simulink model "AFDNFSmodelSPA"  (R2017b)
settings: Solver=ode45  StartTime=0.0  StopTime=1400  FixedStep=1e-3  RelTol=1e-8  EnableMultiTasking=on
PostLoadFcn:
  | run('Methods/NFSOnLoad');
InitFcn:
  | run('Methods/AFDSimInit')
StopFcn:
  | run('Methods/NFSOnLoad');
values from neighbouring files (symbols this model uses):
  nfs = TransferFunction('Plot','true')    [Main.m]    (also in NFSDatabase.sldd = SI
                Imperial
                28184.4409185639)
undefined symbols (not defined in the file or in its folder): Continuous, desired, Earth, F, K_lat, K_long, Kobsvlat, Kobsvlong, lat, latsys, Light, long, longsys, MIL, Newton, Raphson, sigbuilder_block, Time, WGS84
libraries: simulink x6, aerolibtransform2 x2, aerolibwind2 x2, ModelsLibrary x1, ctrlSharedLib x1, sharedutil x1
(part 2 of 4)

== system AFDNFSmodelSPA/Navigation & Sensor System/Navigation Model/01-Test Model/Initialization ==
  Constant4 : Constant  Value=nfs.crusevelvec
  Constant6 : Constant  Value=nfs.angularvel0
  Constant7 : Constant  Value=nfs.attitude0
  Constant8 : Constant  Value=nfs.initialpos
  Reshape{4,6..8} (4 alike) : Reshape  OutputDimensionality=Column vector (2-D)
  Initial Linear Velocity Vector : Outport
  Initial Angular Velocity Vector : Outport  Port=2
  Initial Euler Angles : Outport  Port=3
  Initial Location (NED) : Outport  Port=4
  wires:
  Constant4/1 -> Reshape4/1
  Constant6/1 -> Reshape6/1
  Constant7/1 -> Reshape7/1
  Constant8/1 -> Reshape8/1
  Reshape4/1 -> Initial Linear Velocity Vector/1
  Reshape6/1 -> Initial Angular Velocity Vector/1
  Reshape7/1 -> Initial Euler Angles/1
  Reshape8/1 -> Initial Location (NED)/1

== system AFDNFSmodelSPA/Navigation & Sensor System/Navigation Model/01-Test Model/Navigation Model - Simple ==
  Linear Acceleration (Body) : Inport
  Angular Acceleration (Body) : Inport  Port=2
  Initial Linear Velocity Vector : Inport  Port=3
  Initial Angular Velocity Vector : Inport  Port=4
  Initial Euler Angles : Inport  Port=5
  Initial Location (NED) : Inport  Port=6
  Angular Velocity Integrator (Body) : Integrator  InitialConditionSource=external  InitialCondition=nfs.angularvel0
  Euler angles & Direction Cosine Using Quaternions : Subsystem
  Linear Velocity Integrator (Body) : Integrator  InitialConditionSource=external  InitialCondition=nfs.crusevelvec  ContinuousStateAttributes='BodyVelocity'
  Saturation1 : Saturate  UpperLimit=500  LowerLimit=-500
  Saturation2 : Saturate  UpperLimit=500  LowerLimit=-500
  Linear Velocity (Body) Measured : Outport
  Angular Velocity (Body) Measured : Outport  Port=2
  Euler Angles Measured : Outport  Port=3
  Position (NED) Measured : Outport  Port=4
  Velocity (NED) Measured : Outport  Port=5
  T_BI Measured : Outport  Port=6
  wires:
  Initial Euler Angles/1 -> Euler angles & Direction Cosine Using Quaternions/2(Initial Euler Angles)
  Initial Location (NED)/1 -> Euler angles & Direction Cosine Using Quaternions/3(Initial Location (NED))
  Linear Acceleration (Body)/1 -> Linear Velocity Integrator (Body)/1
  Euler angles & Direction Cosine Using Quaternions/1(Direction Cosine Matrix (T_BI)) -> T_BI Measured/1
  Euler angles & Direction Cosine Using Quaternions/2(Euler Angles) -> Euler Angles Measured/1
  Euler angles & Direction Cosine Using Quaternions/4(Velocity (NED)) -> Velocity (NED) Measured/1
  Saturation1/1 -> Euler angles & Direction Cosine Using Quaternions/1(Linear Velocity), Linear Velocity (Body) Measured/1
  Angular Acceleration (Body)/1 -> Angular Velocity Integrator (Body)/1
  Initial Linear Velocity Vector/1 -> Linear Velocity Integrator (Body)/2
  Euler angles & Direction Cosine Using Quaternions/3(Position (NED)) -> Position (NED) Measured/1
  Linear Velocity Integrator (Body)/1 -> Saturation1/1  "uvw"
  Angular Velocity Integrator (Body)/1 -> Saturation2/1  "pqr"
  Saturation2/1 -> Euler angles & Direction Cosine Using Quaternions/4(Angular Velocities), Angular Velocity (Body) Measured/1
  Initial Angular Velocity Vector/1 -> Angular Velocity Integrator (Body)/2

== system AFDNFSmodelSPA/Nonlinear Flight Simulator/6DoF Nonlinear Flight Equations of Motion (Rigid Body)/AngularAcceleration(Omegadot)/Cross Product ==
  A : Inport
  B : Inport  Port=2
  "A " : InportShadow
  "B " : InportShadow  Port=2
  Subsystem2 : Subsystem
  Subsystem3 : Subsystem
  Sum : Sum  Inputs=+|-  SaturateOnIntegerOverflow=on  InputSameDT=on  OutDataTypeStr=Inherit: Same as first input
  C : Outport
  wires:
  Subsystem3/1(Out2) -> Sum/2
  Subsystem2/1(Out1) -> Sum/1
  A/1 -> Subsystem2/1(A)
  B/1 -> Subsystem2/2(B)
  Sum/1 -> C/1
  "A "/1 -> Subsystem3/1(A)
  "B "/1 -> Subsystem3/2(B)

== system AFDNFSmodelSPA/Nonlinear Flight Simulator/6DoF Nonlinear Flight Equations of Motion (Rigid Body)/Euler angles & Direction Cosine/Euler angles Calculation ==
  Angular Velocities : Inport  PortDimensions=[3,1]
  Euler Angles : Inport  Port=2
  Mux1 : Mux  Inputs=[3 3 3]
  Mux2 : Mux  Inputs=3
  phidot : Fcn  Expr=u[1]+(u[2]*u[4]+u[3]*u[7])*(u[5]/u[8])
  psidot : Fcn  Expr=(u[2]*u[4]+u[3]*u[7])/u[8]
  sincos : Trigonometry  Operator=sincos
  thetadot : Fcn  Expr=u[2]*u[7]-u[3]*u[4]
  Euler Rates : Outport  PortDimensions=[3,1]  InitialOutput=0
  wires:
  sincos/2 -> Mux1/3
  sincos/1 -> Mux1/2
  Mux2/1 -> Euler Rates/1
  phidot/1 -> Mux2/1
  thetadot/1 -> Mux2/2
  psidot/1 -> Mux2/3
  Euler Angles/1 -> sincos/1
  Angular Velocities/1 -> Mux1/1
  Mux1/1 -> psidot/1, phidot/1, thetadot/1

== system AFDNFSmodelSPA/Nonlinear Flight Simulator/6DoF Nonlinear Flight Equations of Motion (Rigid Body)/Euler angles & Direction Cosine/If Action Subsystem ==
  Simulation Termination : Inport
  Action Port : ActionPort  ActionType=then
  Stop Simulation : Stop
  wires:
  Simulation Termination/1 -> Stop Simulation/1

== system AFDNFSmodelSPA/Nonlinear Flight Simulator/6DoF Nonlinear Flight Equations of Motion (Rigid Body)/Euler angles & Direction Cosine/Rotation Angles to DCM ==
  "[R1,R2,R3]" : Inport  PortDimensions=3
  Create 3x3 Matrix : sharedutil/Create 3x3 Matrix
  Fcn11 : Fcn  Expr=u(5)*u(4)
  Fcn12 : Fcn  Expr=u(5)*u(1)
  Fcn13 : Fcn  Expr=-u(2)
  Fcn21 : Fcn  Expr=u(3)*u(2)*u(4) - u(6)*u(1)
  Fcn22 : Fcn  Expr=u(3)*u(2)*u(1) + u(6)*u(4)
  Fcn23 : Fcn  Expr=u(3)*u(5)
  Fcn31 : Fcn  Expr=u(6)*u(2)*u(4) + u(3)*u(1)
  Fcn32 : Fcn  Expr=u(6)*u(2)*u(1) - u(3)*u(4)
  Fcn33 : Fcn  Expr=u(6)*u(5)
  Mux : Mux  Inputs=2
  sincos1 : Trigonometry  Operator=sincos
  DCM : Outport  PortDimensions=[3,3]
  wires:
  "[R1,R2,R3]"/1 -> sincos1/1
  Create 3x3 Matrix/1 -> DCM/1
  sincos1/1 -> Mux/1
  sincos1/2 -> Mux/2
  Mux/1 -> Fcn32/1, Fcn33/1, Fcn31/1, Fcn23/1, Fcn22/1, Fcn11/1, Fcn12/1, Fcn13/1, Fcn21/1
  Fcn11/1 -> Create 3x3 Matrix/1
  Fcn12/1 -> Create 3x3 Matrix/2
  Fcn13/1 -> Create 3x3 Matrix/3
  Fcn21/1 -> Create 3x3 Matrix/4
  Fcn31/1 -> Create 3x3 Matrix/7
  Fcn22/1 -> Create 3x3 Matrix/5
  Fcn23/1 -> Create 3x3 Matrix/6
  Fcn32/1 -> Create 3x3 Matrix/8
  Fcn33/1 -> Create 3x3 Matrix/9

== system AFDNFSmodelSPA/Nonlinear Flight Simulator/6DoF Nonlinear Flight Equations of Motion (Rigid Body)/Euler angles & Direction Cosine/Transform from Body to Inertial axes ==
  Transformation Matrix : Inport
  Position Vector : Inport  Port=2
  Product : Product  Multiplication=Matrix(*)  SaturateOnIntegerOverflow=on  InputSameDT=on  OutDataTypeStr=Inherit: Same as first input
  Reshape1 : Reshape  OutputDimensionality=Column vector (2-D)
  Reshape2 : Reshape
  Ve : Outport
  wires:
  Reshape2/1 -> Ve/1
  Reshape1/1 -> Product/2
  Position Vector/1 -> Reshape1/1
  Transformation Matrix/1 -> Product/1
  Product/1 -> Reshape2/1

== system AFDNFSmodelSPA/Nonlinear Flight Simulator/6DoF Nonlinear Flight Equations of Motion (Rigid Body)/Linear Acceleration(Vdot)/Cross Product ==
  A : Inport
  B : Inport  Port=2
  "A " : InportShadow
  "B " : InportShadow  Port=2
  Subsystem2 : Subsystem
  Subsystem3 : Subsystem
  Sum : Sum  Inputs=+|-  SaturateOnIntegerOverflow=on  InputSameDT=on  OutDataTypeStr=Inherit: Same as first input
  C : Outport
  wires:
  Subsystem3/1(Out2) -> Sum/2
  Subsystem2/1(Out1) -> Sum/1
  A/1 -> Subsystem2/1(A)
  B/1 -> Subsystem2/2(B)
  Sum/1 -> C/1
  "A "/1 -> Subsystem3/1(A)
  "B "/1 -> Subsystem3/2(B)

== system AFDNFSmodelSPA/Nonlinear Flight Simulator/Forces and Moments/Aerodynamic Forces and /Aero Attributes ==
  Linear Velocity (Body) : Inport  PortDimensions=[3,1]
  Altitude : Inport  Port=2
  Beta Saturation : Saturate  UpperLimit=5*pi/11  LowerLimit=-5*pi/11
  Beta Saturation1 : Saturate  UpperLimit=1  LowerLimit=-1
  Demux1 : Demux  Outputs=3
  Derivative1 : Derivative
  Derivative2 : Derivative
  Dynamic Pressure Calc : Subsystem
  Gain : Gain  Gain=0
  Gain1 : Gain
  Linear Velocity (Body)1 : InportShadow  PortDimensions=[3,1]
  Reshape13 : Reshape
  Scope : Scope
  Subsystem : Subsystem
  Trigonometric Function2 : Trigonometry  Operator=atan
  Trigonometric Function3 : Trigonometry  Operator=asin
  Velocity Magnitude : Subsystem
  w/u1 : Product  Inputs=/*  SaturateOnIntegerOverflow=on  InputSameDT=on  OutDataTypeStr=Inherit: Same as first input
  w/u2 : Product  Inputs=*/  SaturateOnIntegerOverflow=on  InputSameDT=on  OutDataTypeStr=Inherit: Same as first input
  w/u3 : Product  Inputs=*/  SaturateOnIntegerOverflow=on  InputSameDT=on  OutDataTypeStr=Inherit: Same as first input
  Alpha : Outport
  Beta : Outport  Port=2
  Dynamic Pressure : Outport  Port=3
  Alphadot : Outport  Port=4
  Betadot : Outport  Port=5
  Mach : Outport  Port=6
  wires:
  Beta Saturation1/1 -> Gain1/1
  Subsystem/2(Air Density) -> Dynamic Pressure Calc/1(Air Density)
  Subsystem/1(Speed of Sound) -> w/u3/2
  Velocity Magnitude/1(Velocity Magnitude) -> w/u3/1, w/u2/2
  Reshape13/1 -> Mach/1
  Derivative2/1 -> Gain/1  "Betadot"
  Beta Saturation/1 -> Beta/1
  Derivative1/1 -> Beta Saturation1/1
  Dynamic Pressure Calc/1(Dynamic Pressure) -> Dynamic Pressure/1
  Linear Velocity (Body)1/1 -> Dynamic Pressure Calc/2(Linear Velocity (Body))
  Altitude/1 -> Subsystem/1(Height)
  w/u3/1 -> Reshape13/1
  Trigonometric Function3/1 -> Beta Saturation/1, Derivative2/1
  Trigonometric Function2/1 -> Derivative1/1, Scope/1, Alpha/1
  w/u2/1 -> Trigonometric Function3/1
  w/u1/1 -> Trigonometric Function2/1
  Demux1/3 -> w/u1/2  "W"
  Demux1/2 -> w/u2/1  "V"
  Demux1/1 -> w/u1/1  "U"
  Linear Velocity (Body)/1 -> Velocity Magnitude/1(Velocity), Demux1/1
  Gain/1 -> Betadot/1
  Gain1/1 -> Alphadot/1

== system AFDNFSmodelSPA/Nonlinear Flight Simulator/Forces and Moments/Aerodynamic Forces and /Energy Analysis1 ==
  Dynamic Pressure : Inport
  Control : Inport  Port=2
  Linear Vel Body : Inport  Port=3
  Angular Vel Body : Inport  Port=4
  Alpha : Inport  Port=5
  Alpha_dot : Inport  Port=6
  Beta : Inport  Port=7
  Beta_dot : Inport  Port=8
  Angular Vel Body0 : InportShadow  Port=4
  Constant{1..2,5,8} (4 alike) : Constant  Value=0
  Constant3 : Constant  Value=ae.refarea
  Constant4 : Constant  Value=ae.span
  Constant6 : Constant  Value=ae.refarea
  Constant9 : Constant  Value=ae.meanchord
  Control3 : InportShadow  Port=2
  Demux1 : Demux
  Demux2 : Demux
  Dynamic Pressure2 : InportShadow
  Lateral-Directional1 : Subsystem
  Linear Vel Body2 : InportShadow  Port=3
  Longitudinal1 : Subsystem
  Lift : Outport
  Drag : Outport  Port=2
  Y Moment : Outport  Port=3
  Side Force : Outport  Port=4
  X Moment : Outport  Port=5
  Z Moment : Outport  Port=6
  wires:
  Lateral-Directional1/1(fy) -> Side Force/1
  Lateral-Directional1/2(l) -> X Moment/1
  Lateral-Directional1/3(n) -> Z Moment/1
  Longitudinal1/2(m) -> Y Moment/1
  Longitudinal1/1(D) -> Drag/1
  Longitudinal1/3(L) -> Lift/1
  Dynamic Pressure/1 -> Lateral-Directional1/1(Dynamic Pressure)
  Constant3/1 -> Lateral-Directional1/2(S)
  Linear Vel Body/1 -> Lateral-Directional1/4(Linear Vel Body)
  Angular Vel Body0/1 -> Lateral-Directional1/5(Angular Vel Body)
  Constant5/1 -> Lateral-Directional1/13(iH)
  Constant4/1 -> Lateral-Directional1/3(b)
  Beta/1 -> Lateral-Directional1/6(Beta)
  Beta_dot/1 -> Lateral-Directional1/7(Beta_dot)
  Demux1/1 -> Lateral-Directional1/8(DeltaElevator)
  Demux1/2 -> Lateral-Directional1/9(DeltaFlap)
  Demux1/4 -> Lateral-Directional1/11(DeltaRudder)
  Demux1/3 -> Lateral-Directional1/10(DeltaAileron)
  Constant1/1 -> Lateral-Directional1/12(DeltaThrust)
  Control/1 -> Demux1/1
  Constant6/1 -> Longitudinal1/2(S)
  Alpha/1 -> Longitudinal1/6(Alpha)
  Angular Vel Body/1 -> Longitudinal1/4(Angular Vel)
  Dynamic Pressure2/1 -> Longitudinal1/1(Dynamic Pressure)
  Linear Vel Body2/1 -> Longitudinal1/3(Linear Vel Body)
  Constant9/1 -> Longitudinal1/5(c_bar)
  Alpha_dot/1 -> Longitudinal1/7(Alpha_dot)
  Constant8/1 -> Longitudinal1/13(iH)
  Constant2/1 -> Longitudinal1/12(Delta_Thrust)
  Demux2/4 -> Longitudinal1/11(DeltaRudder)
  Demux2/2 -> Longitudinal1/9(DeltaFlap)
  Demux2/3 -> Longitudinal1/10(DeltaAileron)
  Demux2/1 -> Longitudinal1/8(DeltaElevator)
  Control3/1 -> Demux2/1

== system AFDNFSmodelSPA/Nonlinear Flight Simulator/Forces and Moments/Aerodynamic Forces and /Forces ==
  Linear Velocity : Inport  PortDimensions=[3,1]
  Alpha : Inport  Port=2  PortDimensions=1
  Beta : Inport  Port=3
  Angular Velocity : Inport  Port=4  PortDimensions=[3,1]
  Control : Inport  Port=5  PortDimensions=[4,1]
  Dynamic Pressure : Inport  Port=6  PortDimensions=[1,1]
  Alphadot : Inport  Port=7  PortDimensions=1
  Mach : Inport  Port=8
  Aerodynamic Forces : Subsystem
  Alpha1 : InportShadow  Port=2  PortDimensions=1
  Beta1 : InportShadow  Port=3
  Force Coefficients Calculator : Subsystem
  Aerodynamic Forces (Body) : Outport
  wires:
  Aerodynamic Forces/1(Aerodynamic Forces) -> Aerodynamic Forces (Body)/1
  Control/1 -> Force Coefficients Calculator/5(Control)
  Angular Velocity/1 -> Force Coefficients Calculator/4(Angular Velocity)
  Alphadot/1 -> Force Coefficients Calculator/6(Alphadot)
  Mach/1 -> Force Coefficients Calculator/7(Mach)
  Linear Velocity/1 -> Force Coefficients Calculator/1(Linear Velocity)
  Alpha/1 -> Force Coefficients Calculator/2(Alpha)
  Beta/1 -> Force Coefficients Calculator/3(Beta)
  Force Coefficients Calculator/1(CL) -> Aerodynamic Forces/1(CL)
  Force Coefficients Calculator/2(CD) -> Aerodynamic Forces/2(CD)
  Force Coefficients Calculator/3(CY) -> Aerodynamic Forces/3(CY)
  Alpha1/1 -> Aerodynamic Forces/5(Alpha)
  Dynamic Pressure/1 -> Aerodynamic Forces/4(Dynamic Pressure)
  Beta1/1 -> Aerodynamic Forces/6(Beta)

== system AFDNFSmodelSPA/Nonlinear Flight Simulator/Forces and Moments/Aerodynamic Forces and /Moments ==
  Linear Velocity : Inport  PortDimensions=[3,1]
  Alpha : Inport  Port=2
  Beta : Inport  Port=3
  Angular Velocity : Inport  Port=4  PortDimensions=[3,1]
  Control : Inport  Port=5
  Dynamic Pressure : Inport  Port=6
  Alphadot : Inport  Port=7
  Mach : Inport  Port=8
  "Aerodynamic Moment " : Subsystem
  Alpha1 : InportShadow  Port=2
  Beta1 : InportShadow  Port=3
  Beta2 : InportShadow  Port=3
  Demux1 : Demux  Outputs=3
  Demux2 : Demux
  Linear Velocity1 : InportShadow  PortDimensions=[3,1]
  Linear Velocity2 : InportShadow  PortDimensions=[3,1]
  Pitch Moment Coefficient : Subsystem
  Roll Moment Coefficient : Subsystem
  Yaw Moment Coefficient : Subsystem
  Aerodynamic Moments (Body) : Outport
  wires:
  Demux2/2 -> Pitch Moment Coefficient/5(DeltaFlap)
  Demux2/1 -> Pitch Moment Coefficient/4(DeltaElevator)
  Demux2/4 -> Yaw Moment Coefficient/6(DeltaRudder), Roll Moment Coefficient/6(DeltaRudder)
  Demux2/3 -> Yaw Moment Coefficient/5(DeltaAileron), Roll Moment Coefficient/5(DeltaAileron)
  Control/1 -> Demux2/1
  Mach/1 -> Pitch Moment Coefficient/7(Mach)
  Alphadot/1 -> Pitch Moment Coefficient/6(Alphadot)
  Demux1/2 -> Pitch Moment Coefficient/3(Q)
  Demux1/3 -> Yaw Moment Coefficient/4(R), Roll Moment Coefficient/4(R)
  Demux1/1 -> Yaw Moment Coefficient/3(P), Roll Moment Coefficient/3(P)
  Angular Velocity/1 -> Demux1/1
  Beta1/1 -> Yaw Moment Coefficient/2(beta)
  Beta/1 -> Roll Moment Coefficient/2(Beta)
  Alpha/1 -> Pitch Moment Coefficient/2(Alpha)
  Dynamic Pressure/1 -> "Aerodynamic Moment "/4(Dynamic Pressure)
  Linear Velocity2/1 -> Yaw Moment Coefficient/1(Linear Velocity)
  Linear Velocity1/1 -> Pitch Moment Coefficient/1(Linear Velocity)
  Linear Velocity/1 -> Roll Moment Coefficient/1(Linear Velocity)
  "Aerodynamic Moment "/1(Aerodynamic Moments) -> Aerodynamic Moments (Body)/1
  Yaw Moment Coefficient/1(Cn) -> "Aerodynamic Moment "/3(Cn)
  Pitch Moment Coefficient/1(Cm) -> "Aerodynamic Moment "/2(Cm)
  Roll Moment Coefficient/1(Cl) -> "Aerodynamic Moment "/1(Cl)
  Alpha1/1 -> "Aerodynamic Moment "/5(Alpha)
  Beta2/1 -> "Aerodynamic Moment "/6(Beta)

== system AFDNFSmodelSPA/Nonlinear Flight Simulator/Forces and Moments/Aerodynamic Forces and /Turbulence ==
  Linear Velocity : Inport  PortDimensions=[3,1]
  Angular Velocity : Inport  Port=2  PortDimensions=[3,1]
  Altitude : Inport  Port=3  PortDimensions=1
  DCM : Inport  Port=4  PortDimensions=[3,3]
  Bus Creator : BusCreator  Inputs=4
  Turbulence Model : Subsystem  Variant=on
  Turbulent Velocity : Outport
  wires:
  Linear Velocity/1 -> Bus Creator/1  "Linear Velocity"
  Altitude/1 -> Bus Creator/3  "Altitude"
  DCM/1 -> Bus Creator/4  "DCM"
  Bus Creator/1 -> Turbulence Model/1(In)
  Angular Velocity/1 -> Bus Creator/2  "Angular Velocity"
  Turbulence Model/1(Out) -> Turbulent Velocity/1

== system AFDNFSmodelSPA/Nonlinear Flight Simulator/Forces and Moments/Thrust/Signal Builder ==
  Demux : Demux  Tag=STV Demux  Outputs=1
  FromWs : FromWorkspace  Tag=STV FromWs  VariableName=tuvar  SampleTime=0
      SigBuilderData=|
      | common.afterFinalStr = 'Extrapolate'
      | common.sampleTime = 0
      | dataSet.timeRange = [0 1200]
      | dataSet.name = 'Thrust Deviation'
      | sbobj.Groups.Name = 'Thrust Deviation'
      | sbobj.Groups.Signals.Name = 'ThrustDeviation'
      | sbobj.Groups.Signals.XData = [0 10 10 12 12 1200]
      | sbobj.Groups.Signals.YData = [1 1 1.05 1.05 1 1]
      | sbobj.Groups.TimeRange = [0 1200]
  ThrustDeviation : Outport  Tag=STV Outport
  wires:
  Demux/1 -> ThrustDeviation/1
  FromWs/1 -> Demux/1

== system AFDNFSmodelSPA/Nonlinear Flight Simulator/Forces and Moments/Weight/Vector Magnitude ==
  Vector : Inport
  Dot Product : DotProduct  InputSameDT=on  OutDataTypeStr=Inherit: Inherit via internal rule
  Sqrt : Sqrt  SaturateOnIntegerOverflow=on
  Vector Magnitude : Outport
  wires:
  Sqrt/1 -> Vector Magnitude/1  "abs(V)"
  Vector/1 -> Dot Product/2, Dot Product/1
  Dot Product/1 -> Sqrt/1

== system AFDNFSmodelSPA/Nonlinear Flight Simulator/Plot/Cockpit Monitors/Airspeed Indicator ==

== system AFDNFSmodelSPA/OnBoardComputer/Control System/Trim Offset + Reference Excitation/Doublet Generated Signal ==
  Constant : Constant  Value=[0;0;0]
  Constant2 : Constant  Value=nfs.trim.delta_e
  Doublet : Subsystem  mask{T_start=10, amp=deg2rad(2), span=1, sampletime=0}
      mask prompts: T_start "Doublet Time"; amp "Amplitude"; span "Time Span"; sampletime "Sample Time"
      mask Display: plot([0,1,1,2,2,3,3,4],[0,0,1,1,-1,-1,0,0])
  Mux : Mux  Inputs=2
  Sum : Sum  Inputs=|++
  Doublet Out : Outport
  wires:
  Sum/1 -> Mux/1
  Constant/1 -> Mux/2
  Doublet/1(Out1) -> Sum/1
  Constant2/1 -> Sum/2
  Mux/1 -> Doublet Out/1

== system AFDNFSmodelSPA/OnBoardComputer/Control System/Trim Offset + Reference Excitation/Triangular signal span 10 sec ==
  Constant1 : Constant  Value=0
  Constant2 : Constant  Value=nfs.trim.delta_e
  Constant3 : Constant  Value=0
  Constant4 : Constant  Value=0
  Gain{,1..3} (4 alike) : Gain  Gain=pi/180
  Gain4 : Gain  Gain=0
  Gain5 : Gain  Gain=10
  Gain6 : Gain  Gain=0
  Gain7 : Gain  Gain=0
  Mux : Mux
  Signal Builder1 : Subsystem  Tag=STV Subsys  LoadFcn=sigbuilder_block('load');  StartFcn=sigbuilder_block('start');  StopFcn=sigbuilder_block('stop');  ClipboardFcn=sigbuilder_block('clipboard');  mask(Sigbuilder block){tuvar=[0:10]}
      mask help: Simulink:masks:SigbuilderBlock_MD
      mask init:
      | if ~strcmp(get_param(bdroot(gcbh),'SimulationStatus'),'stopped') tuvar = sigbuilder_block('maskInit'); end
      settings: CopyFcn=sigbuilder_block('copy');  DeleteFcn=sigbuilder_block('delete');  ModelCloseFcn=sigbuilder_block('modelClose');  PreSaveFcn=sigbuilder_block('preSave');  PauseFcn=sigbuilder_block('pause');  ContinueFcn=sigbuilder_block('continue');  NameChangeFcn=sigbuilder_block('namechange');  OpenFcn=sigbuilder_block('open',[437.4 199.2 550.2 400.2 ]);  CloseFcn=sigbuilder_block('close');
      mask Display: plot(0, 0, 100, 100,[2, 2, 32, 32, 2], [68, 8, 8, 68, 68],[32, 2], [38, 38], [32, 19, 2],[53, 60, 44], [32, 17, 17, 2],[16, 16, 31, 31]);txt = getActiveGroup(gcbh);text(2, 100, txt,'verticalAlignment', 'top');
  Signal Builder2 : Subsystem  Tag=STV Subsys  LoadFcn=sigbuilder_block('load');  StartFcn=sigbuilder_block('start');  StopFcn=sigbuilder_block('stop');  ClipboardFcn=sigbuilder_block('clipboard');  mask(Sigbuilder block){tuvar=[0:10]}
      mask help: Simulink:masks:SigbuilderBlock_MD
      mask init:
      | if ~strcmp(get_param(bdroot(gcbh),'SimulationStatus'),'stopped') tuvar = sigbuilder_block('maskInit'); end
      settings: CopyFcn=sigbuilder_block('copy');  DeleteFcn=sigbuilder_block('delete');  ModelCloseFcn=sigbuilder_block('modelClose');  PreSaveFcn=sigbuilder_block('preSave');  PauseFcn=sigbuilder_block('pause');  ContinueFcn=sigbuilder_block('continue');  NameChangeFcn=sigbuilder_block('namechange');  OpenFcn=sigbuilder_block('open',[437.25 199.5 550.5 399.75 ]);  CloseFcn=sigbuilder_block('close');
      mask Display: plot(0, 0, 100, 100,[2, 2, 32, 32, 2], [68, 8, 8, 68, 68],[32, 2], [38, 38], [32, 19, 2],[53, 60, 44], [32, 17, 17, 2],[16, 16, 31, 31]);txt = getActiveGroup(gcbh);text(2, 100, txt,'verticalAlignment', 'top');
  Signal Builder3 : Subsystem  Tag=STV Subsys  LoadFcn=sigbuilder_block('load');  StartFcn=sigbuilder_block('start');  StopFcn=sigbuilder_block('stop');  ClipboardFcn=sigbuilder_block('clipboard');  mask(Sigbuilder block){tuvar=[0:10]}
      mask help: Simulink:masks:SigbuilderBlock_MD
      mask init:
      | if ~strcmp(get_param(bdroot(gcbh),'SimulationStatus'),'stopped') tuvar = sigbuilder_block('maskInit'); end
      settings: CopyFcn=sigbuilder_block('copy');  DeleteFcn=sigbuilder_block('delete');  ModelCloseFcn=sigbuilder_block('modelClose');  PreSaveFcn=sigbuilder_block('preSave');  PauseFcn=sigbuilder_block('pause');  ContinueFcn=sigbuilder_block('continue');  NameChangeFcn=sigbuilder_block('namechange');  OpenFcn=sigbuilder_block('open',[437.4 199.2 550.2 400.2 ]);  CloseFcn=sigbuilder_block('close');
      mask Display: plot(0, 0, 100, 100,[2, 2, 32, 32, 2], [68, 8, 8, 68, 68],[32, 2], [38, 38], [32, 19, 2],[53, 60, 44], [32, 17, 17, 2],[16, 16, 31, 31]);txt = getActiveGroup(gcbh);text(2, 100, txt,'verticalAlignment', 'top');
  Signal Builder4 : Subsystem  Tag=STV Subsys  LoadFcn=sigbuilder_block('load');  StartFcn=sigbuilder_block('start');  StopFcn=sigbuilder_block('stop');  ClipboardFcn=sigbuilder_block('clipboard');  mask(Sigbuilder block){tuvar=[0:10]}
      mask help: Simulink:masks:SigbuilderBlock_MD
      mask init:
      | if ~strcmp(get_param(bdroot(gcbh),'SimulationStatus'),'stopped') tuvar = sigbuilder_block('maskInit'); end
      settings: CopyFcn=sigbuilder_block('copy');  DeleteFcn=sigbuilder_block('delete');  ModelCloseFcn=sigbuilder_block('modelClose');  PreSaveFcn=sigbuilder_block('preSave');  PauseFcn=sigbuilder_block('pause');  ContinueFcn=sigbuilder_block('continue');  NameChangeFcn=sigbuilder_block('namechange');  OpenFcn=sigbuilder_block('open',[437.4 199.2 550.2 400.2 ]);  CloseFcn=sigbuilder_block('close');
      mask Display: plot(0, 0, 100, 100,[2, 2, 32, 32, 2], [68, 8, 8, 68, 68],[32, 2], [38, 38], [32, 19, 2],[53, 60, 44], [32, 17, 17, 2],[16, 16, 31, 31]);txt = getActiveGroup(gcbh);text(2, 100, txt,'verticalAlignment', 'top');
  Sum{,1..3} (4 alike) : Sum  Inputs=++|
  Tri : Outport
  wires:
  Mux/1 -> Tri/1
  Signal Builder1/1(Normalized Elevator(deg)) -> Gain/1
  Constant2/1 -> Sum/1
  Gain/1 -> Sum/2
  Signal Builder2/1(Normalized Flap(deg)) -> Gain1/1
  Constant1/1 -> Sum1/1
  Gain1/1 -> Sum1/2
  Signal Builder3/1(Normalized Alileron(deg)) -> Gain2/1
  Constant3/1 -> Sum2/1
  Gain2/1 -> Sum2/2
  Signal Builder4/1(Normalized Rudder(deg)) -> Gain3/1
  Constant4/1 -> Sum3/1
  Gain3/1 -> Sum3/2
  Sum/1 -> Gain7/1
  Sum1/1 -> Gain6/1
  Sum2/1 -> Gain5/1
  Sum3/1 -> Gain4/1
  Gain4/1 -> Mux/4
  Gain5/1 -> Mux/3
  Gain6/1 -> Mux/2
  Gain7/1 -> Mux/1

== system AFDNFSmodelSPA/OnBoardComputer/Control System/Unfinished Controllers (State-Feedback)/Full-State Feedback Servo ==
  States : Inport
  Gain : Gain  Gain=-K_long  Multiplication=Matrix(K*u) (u vector)
  Gain1 : Gain  Gain=-K_lat  Multiplication=Matrix(K*u) (u vector)
  Selector1 : Selector  InputPortWidth=9  IndexOptions=Index vector (dialog)  Indices=[5:9]  OutputSizes=1
  Selector3 : Selector  InputPortWidth=9  IndexOptions=Index vector (dialog)  Indices=[1:4]  OutputSizes=1
  Longitudinal Control : Outport
  Lateral-Directional Control : Outport  Port=2
  wires:
  Gain1/1 -> Lateral-Directional Control/1
  Gain/1 -> Longitudinal Control/1
  Selector1/1 -> Gain1/1  "Lateral-Directional"
  Selector3/1 -> Gain/1  "Longitudinal"
  States/1 -> Selector1/1, Selector3/1

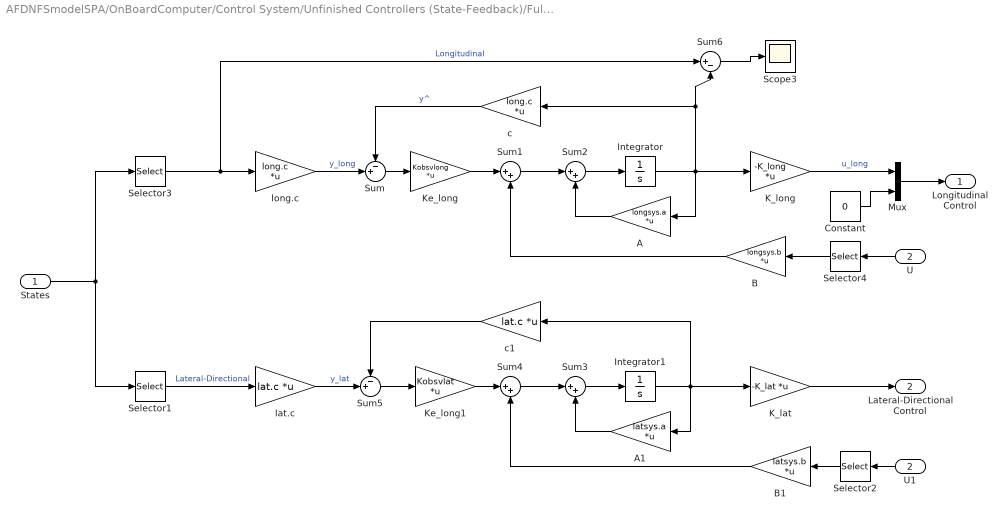
== system AFDNFSmodelSPA/OnBoardComputer/Control System/Unfinished Controllers (State-Feedback)/Full-State Observer Servo ==
  States : Inport  PortDimensions=[9,1]
  U : Inport  Port=2  PortDimensions=[4,1]
  A : Gain  Gain=longsys.a  Multiplication=Matrix(K*u)
  A1 : Gain  Gain=latsys.a  Multiplication=Matrix(K*u)
  B : Gain  Gain=longsys.b  Multiplication=Matrix(K*u)
  B1 : Gain  Gain=latsys.b  Multiplication=Matrix(K*u)
  Constant : Constant  Value=0
  Integrator : Integrator
  Integrator1 : Integrator
  K_lat : Gain  Gain=-K_lat  Multiplication=Matrix(K*u)
  K_long : Gain  Gain=-K_long  Multiplication=Matrix(K*u)
  Ke_long : Gain  Gain=Kobsvlong  Multiplication=Matrix(K*u)
  Ke_long1 : Gain  Gain=Kobsvlat  Multiplication=Matrix(K*u)
  Mux : Mux  Inputs=2
  Scope3 : Scope
  Selector1 : Selector  InputPortWidth=9  IndexOptions=Index vector (dialog)  Indices=[5:9]  OutputSizes=1
  Selector2 : Selector  InputPortWidth=4  IndexOptions=Index vector (dialog)  Indices=[3:4]  OutputSizes=1
  Selector3 : Selector  InputPortWidth=9  IndexOptions=Index vector (dialog)  Indices=[1:4]  OutputSizes=1
  Selector4 : Selector  InputPortWidth=4  IndexOptions=Index vector (dialog)  Indices=[1]  OutputSizes=1
  Sum : Sum  Inputs=-+|
  Sum{1..4} (4 alike) : Sum  Inputs=|++
  Sum5 : Sum  Inputs=-+|
  Sum6 : Sum  Inputs=|+-
  U1 : InportShadow  Port=2  PortDimensions=[4,1]
  c : Gain  Gain=long.c  Multiplication=Matrix(K*u)
  c1 : Gain  Gain=lat.c  Multiplication=Matrix(K*u)
  lat.c : Gain  Gain=lat.c  Multiplication=Matrix(K*u)
  long.c : Gain  Gain=long.c  Multiplication=Matrix(K*u)
  Longitudinal Control : Outport
  Lateral-Directional Control : Outport  Port=2
  wires:
  Constant/1 -> Mux/2
  K_long/1 -> Mux/1  "u_long"
  Mux/1 -> Longitudinal Control/1
  Selector2/1 -> B1/1
  Selector4/1 -> B/1
  U1/1 -> Selector2/1
  U/1 -> Selector4/1
  Sum6/1 -> Scope3/1
  c1/1 -> Sum5/1
  B1/1 -> Sum4/2
  A1/1 -> Sum3/2
  Sum3/1 -> Integrator1/1
  Sum4/1 -> Sum3/1
  Ke_long1/1 -> Sum4/1
  Sum5/1 -> Ke_long1/1
  lat.c/1 -> Sum5/2  "y_lat"
  Integrator1/1 -> c1/1, A1/1, K_lat/1
  c/1 -> Sum/1  "y^"
  long.c/1 -> Sum/2  "y_long"
  A/1 -> Sum2/2
  Integrator/1 -> Sum6/2, c/1, K_long/1, A/1
  Sum2/1 -> Integrator/1
  Sum1/1 -> Sum2/1
  B/1 -> Sum1/2
  Ke_long/1 -> Sum1/1
  Sum/1 -> Ke_long/1
  States/1 -> Selector3/1, Selector1/1
  Selector3/1 -> Sum6/1, long.c/1  "Longitudinal"
  Selector1/1 -> lat.c/1  "Lateral-Directional"
  K_lat/1 -> Lateral-Directional Control/1

== system AFDNFSmodelSPA/OnBoardComputer/Control System/Unfinished Controllers (State-Feedback)/Reduced Order Observer Servo ==
  States : Inport  PortDimensions=[9,1]
  A : Gain  Gain=longsys.a  Multiplication=Matrix(K*u)
  A1 : Gain  Gain=latsys.a  Multiplication=Matrix(K*u)
  B : Gain  Gain=longsys.b  Multiplication=Matrix(K*u)
  B1 : Gain  Gain=latsys.b  Multiplication=Matrix(K*u)
  Integrator : Integrator
  Integrator1 : Integrator
  K_lat : Gain  Gain=-K_lat  Multiplication=Matrix(K*u)
  K_long : Gain  Gain=-K_long  Multiplication=Matrix(K*u)
  Ke_long : Gain  Gain=Kobsvlong  Multiplication=Matrix(K*u)
  Ke_long1 : Gain  Gain=Kobsvlat  Multiplication=Matrix(K*u)
  Selector1 : Selector  InputPortWidth=9  IndexOptions=Index vector (dialog)  Indices=[5:9]  OutputSizes=1
  Selector3 : Selector  InputPortWidth=9  IndexOptions=Index vector (dialog)  Indices=[1:4]  OutputSizes=1
  Sum : Sum  Inputs=-+|
  Sum1 : Sum  Inputs=|++
  Sum2 : Sum  Inputs=|+-
  Sum3 : Sum  Inputs=|+-
  Sum4 : Sum  Inputs=|++
  Sum5 : Sum  Inputs=-+|
  c : Gain  Gain=long.c  Multiplication=Matrix(K*u)
  c1 : Gain  Gain=lat.c  Multiplication=Matrix(K*u)
  lat.c : Gain  Gain=lat.c  Multiplication=Matrix(K*u)
  long.c : Gain  Gain=long.c  Multiplication=Matrix(K*u)
  Longitudinal Control : Outport
  Lateral-Directional Control : Outport  Port=2
  wires:
  K_lat/1 -> Lateral-Directional Control/1, B1/1
  K_long/1 -> Longitudinal Control/1, B/1  "u_long"
  Selector1/1 -> lat.c/1  "Lateral-Directional"
  Selector3/1 -> long.c/1  "Longitudinal"
  States/1 -> Selector1/1, Selector3/1
  Sum/1 -> Ke_long/1
  Ke_long/1 -> Sum1/1
  B/1 -> Sum1/2
  Sum1/1 -> Sum2/1
  Sum2/1 -> Integrator/1
  Integrator/1 -> A/1, K_long/1, c/1
  A/1 -> Sum2/2
  long.c/1 -> Sum/2  "y_long"
  c/1 -> Sum/1
  Integrator1/1 -> K_lat/1, A1/1, c1/1
  lat.c/1 -> Sum5/2  "y_lat"
  Sum5/1 -> Ke_long1/1
  Ke_long1/1 -> Sum4/1
  Sum4/1 -> Sum3/1
  Sum3/1 -> Integrator1/1
  A1/1 -> Sum3/2
  B1/1 -> Sum4/2
  c1/1 -> Sum5/1

== system AFDNFSmodelSPA/Navigation & Sensor System/Navigation Model/01-Test Model/Navigation Model - Simple/Euler angles & Direction Cosine Using Quaternions ==
  Linear Velocity : Inport  PortDimensions=[3,1]
  Initial Euler Angles : Inport  Port=2  PortDimensions=[3,1]
  Initial Location (NED) : Inport  Port=3  PortDimensions=[3,1]
  Angular Velocities : Inport  Port=4  PortDimensions=[3,1]
  Constant : Constant
  If : If  IfExpression=u1(3)>= 0  ShowElse=off
  If Action Subsystem : Subsystem  TreatAsAtomicUnit=on
  Position Integrator : Integrator  InitialConditionSource=external  InitialCondition=[0,0,nfs.attitude0]
  Quaternion Rates : Subsystem
  Quaternions Int : Integrator  InitialConditionSource=external  InitialCondition=nfs.attitude0  ContinuousStateAttributes='Quaternions'
  Rotation Angles to DCM1 : Subsystem
  Rotation Angles to Quaternions : Subsystem
  Rotation Angles to Quaternions1 : Subsystem
  Scope : Scope
  Selector3 : Selector  InputPortWidth=3  IndexOptions=Index vector (dialog)  Indices=[3 2 1]  OutputSizes=1
  Selector4 : Selector  InputPortWidth=3  IndexOptions=Index vector (dialog)  Indices=[3 2 1]  OutputSizes=1
  Transform from Body to Inertial axes : Subsystem
      mask Display: disp('T_IB')
  Transpose : Math  Operator=transpose  SaturateOnIntegerOverflow=on
  Direction Cosine Matrix (T_BI) : Outport  PortDimensions=[3,3]
  Euler Angles : Outport  Port=2  PortDimensions=[3,1]
  Position (NED) : Outport  Port=3  PortDimensions=[3,1]
  Velocity (NED) : Outport  Port=4  PortDimensions=[3,1]
  wires:
  Position Integrator/1 -> Position (NED)/1, If/1
  Transform from Body to Inertial axes/1(Ve) -> Position Integrator/1, Velocity (NED)/1
  Initial Location (NED)/1 -> Position Integrator/2
  Linear Velocity/1 -> Transform from Body to Inertial axes/2(Position Vector)
  Transpose/1 -> Transform from Body to Inertial axes/1(Transformation Matrix)
  Quaternion Rates/1(Quaternion Rates) -> Quaternions Int/1
  Angular Velocities/1 -> Quaternion Rates/1(Angular Velocities)
  Initial Euler Angles/1 -> Selector3/1
  Selector3/1 -> Rotation Angles to Quaternions/1("[R1,R2,R3]")
  Rotation Angles to Quaternions/1(Quat) -> Quaternions Int/2
  Quaternions Int/1 -> Quaternion Rates/2(Quaternions), Rotation Angles to Quaternions1/1(q), Rotation Angles to DCM1/1(q)
  Rotation Angles to Quaternions1/1(Quat2RotAngs) -> Selector4/1
  Selector4/1 -> Euler Angles/1, Scope/1
  Rotation Angles to DCM1/1(DCM) -> Direction Cosine Matrix (T_BI)/1, Transpose/1
  Constant/1 -> If Action Subsystem/1(Simulation Termination)
  If/1 -> If Action Subsystem/Action

== system AFDNFSmodelSPA/Nonlinear Flight Simulator/6DoF Nonlinear Flight Equations of Motion (Rigid Body)/AngularAcceleration(Omegadot)/Cross Product/Subsystem2 ==
  A : Inport
  B : Inport  Port=2
  Demux : Demux  Outputs=3
  Demux1 : Demux  Outputs=3
  Mux : Mux  Inputs=3
  i x j : Product  SaturateOnIntegerOverflow=on  InputSameDT=on  OutDataTypeStr=Inherit: Same as first input
  j x k : Product  SaturateOnIntegerOverflow=on  InputSameDT=on  OutDataTypeStr=Inherit: Same as first input
  k x i : Product  SaturateOnIntegerOverflow=on  InputSameDT=on  OutDataTypeStr=Inherit: Same as first input
  Out1 : Outport
  wires:
  Demux1/3 -> j x k/2
  Demux/2 -> j x k/1
  Demux/3 -> k x i/1
  Demux1/1 -> k x i/2
  Demux1/2 -> i x j/2
  Demux/1 -> i x j/1
  i x j/1 -> Mux/3
  k x i/1 -> Mux/2
  j x k/1 -> Mux/1
  B/1 -> Demux1/1
  A/1 -> Demux/1
  Mux/1 -> Out1/1

== system AFDNFSmodelSPA/Nonlinear Flight Simulator/6DoF Nonlinear Flight Equations of Motion (Rigid Body)/AngularAcceleration(Omegadot)/Cross Product/Subsystem3 ==
  A : Inport
  B : Inport  Port=2
  Demux : Demux  Outputs=3
  Demux1 : Demux  Outputs=3
  Mux : Mux  Inputs=3
  i x k : Product  SaturateOnIntegerOverflow=on  InputSameDT=on  OutDataTypeStr=Inherit: Same as first input
  j x i : Product  SaturateOnIntegerOverflow=on  InputSameDT=on  OutDataTypeStr=Inherit: Same as first input
  k x j : Product  SaturateOnIntegerOverflow=on  InputSameDT=on  OutDataTypeStr=Inherit: Same as first input
  Out2 : Outport
  wires:
  j x i/1 -> Mux/3
  i x k/1 -> Mux/2
  k x j/1 -> Mux/1
  Mux/1 -> Out2/1
  Demux1/1 -> j x i/2
  Demux/2 -> j x i/1
  Demux1/3 -> i x k/2
  Demux/1 -> i x k/1
  Demux1/2 -> k x j/2
  Demux/3 -> k x j/1
  B/1 -> Demux1/1
  A/1 -> Demux/1

== system AFDNFSmodelSPA/Nonlinear Flight Simulator/6DoF Nonlinear Flight Equations of Motion (Rigid Body)/Linear Acceleration(Vdot)/Cross Product/Subsystem2 ==
  A : Inport
  B : Inport  Port=2
  Demux : Demux  Outputs=3
  Demux1 : Demux  Outputs=3
  Mux : Mux  Inputs=3
  i x j : Product  SaturateOnIntegerOverflow=on  InputSameDT=on  OutDataTypeStr=Inherit: Same as first input
  j x k : Product  SaturateOnIntegerOverflow=on  InputSameDT=on  OutDataTypeStr=Inherit: Same as first input
  k x i : Product  SaturateOnIntegerOverflow=on  InputSameDT=on  OutDataTypeStr=Inherit: Same as first input
  Out1 : Outport
  wires:
  Demux1/3 -> j x k/2
  Demux/2 -> j x k/1
  Demux/3 -> k x i/1
  Demux1/1 -> k x i/2
  Demux1/2 -> i x j/2
  Demux/1 -> i x j/1
  i x j/1 -> Mux/3
  k x i/1 -> Mux/2
  j x k/1 -> Mux/1
  B/1 -> Demux1/1
  A/1 -> Demux/1
  Mux/1 -> Out1/1

== system AFDNFSmodelSPA/Nonlinear Flight Simulator/6DoF Nonlinear Flight Equations of Motion (Rigid Body)/Linear Acceleration(Vdot)/Cross Product/Subsystem3 ==
  A : Inport
  B : Inport  Port=2
  Demux : Demux  Outputs=3
  Demux1 : Demux  Outputs=3
  Mux : Mux  Inputs=3
  i x k : Product  SaturateOnIntegerOverflow=on  InputSameDT=on  OutDataTypeStr=Inherit: Same as first input
  j x i : Product  SaturateOnIntegerOverflow=on  InputSameDT=on  OutDataTypeStr=Inherit: Same as first input
  k x j : Product  SaturateOnIntegerOverflow=on  InputSameDT=on  OutDataTypeStr=Inherit: Same as first input
  Out2 : Outport
  wires:
  j x i/1 -> Mux/3
  i x k/1 -> Mux/2
  k x j/1 -> Mux/1
  Mux/1 -> Out2/1
  Demux1/1 -> j x i/2
  Demux/2 -> j x i/1
  Demux1/3 -> i x k/2
  Demux/1 -> i x k/1
  Demux1/2 -> k x j/2
  Demux/3 -> k x j/1
  B/1 -> Demux1/1
  A/1 -> Demux/1

== system AFDNFSmodelSPA/Nonlinear Flight Simulator/Forces and Moments/Aerodynamic Forces and /Aero Attributes/Dynamic Pressure Calc ==
  Air Density : Inport  PortDimensions=1
  Linear Velocity (Body) : Inport  Port=2  PortDimensions=[3 1]
  0.5*rh : Product  SaturateOnIntegerOverflow=on  InputSameDT=on  OutDataTypeStr=Inherit: Same as first input
  Dot Product : DotProduct  InputSameDT=on  OutDataTypeStr=Inherit: Inherit via internal rule
  Gain : Gain  Gain=0.5  SaturateOnIntegerOverflow=on  OutDataTypeStr=Inherit: Same as input  ParamDataTypeStr=Inherit: Same as input
  V^2 : Abs
  Dynamic Pressure : Outport
  wires:
  Dot Product/1 -> V^2/1
  Linear Velocity (Body)/1 -> Dot Product/2, Dot Product/1
  Air Density/1 -> Gain/1
  V^2/1 -> 0.5*rh/1
  Gain/1 -> 0.5*rh/2
  0.5*rh/1 -> Dynamic Pressure/1

== system AFDNFSmodelSPA/Nonlinear Flight Simulator/Forces and Moments/Aerodynamic Forces and /Aero Attributes/Subsystem ==
  Height : Inport
  "(T/T0)^(g/LR) " : Math  Operator=pow  SaturateOnIntegerOverflow=on
  1/T0 : Gain  Gain=1/288.15  SaturateOnIntegerOverflow=on  OutDataTypeStr=Inherit: Same as input  ParamDataTypeStr=Inherit: Same as input
  Altitude of Troposphere : Constant  Value=11000  OutDataTypeStr=Inherit: Inherit via back propagation
  Lapse Rate : Gain  Gain=0.0065  SaturateOnIntegerOverflow=on  OutDataTypeStr=Inherit: Same as input  ParamDataTypeStr=Inherit: Same as input
  Limit altitude  to Stratosphere : Saturate  UpperLimit=0  LowerLimit=11000-20000
  Limit altitude  to troposhere : Saturate  UpperLimit=11000  LowerLimit=0
  Product : Product  Inputs=*/  SaturateOnIntegerOverflow=on  InputSameDT=on  OutDataTypeStr=Inherit: Same as first input
  Product1 : Product  Inputs=/*  SaturateOnIntegerOverflow=on  InputSameDT=on  OutDataTypeStr=Inherit: Same as first input
  Product3 : Product  SaturateOnIntegerOverflow=on  InputSameDT=on  OutDataTypeStr=Inherit: Same as first input
  Sea Level Temperature : Constant  Value=288.15  OutDataTypeStr=Inherit: Inherit via back propagation
  Stratosphere Model : Math  SaturateOnIntegerOverflow=on
  Sum : Sum  Inputs=+-  SaturateOnIntegerOverflow=on  InputSameDT=on  OutDataTypeStr=Inherit: Same as first input
  Sum1 : Sum  Inputs=+-  SaturateOnIntegerOverflow=on  InputSameDT=on  OutDataTypeStr=Inherit: Same as first input
  a : Sqrt  AlgorithmType=Newton-Raphson  SaturateOnIntegerOverflow=on
  g/(L*R) : Constant  Value=9.80665/(0.0065*287.0531)  OutDataTypeStr=Inherit: Inherit via back propagation
  g/R : Gain  Gain=9.80665/287.0531  SaturateOnIntegerOverflow=on  OutDataTypeStr=Inherit: Same as input  ParamDataTypeStr=Inherit: Same as input
  gamma*R : Gain  Gain=1.4*287.0531  SaturateOnIntegerOverflow=on  OutDataTypeStr=Inherit: Same as input  ParamDataTypeStr=Inherit: Same as input
  rho0 : Gain  Gain=1.225  SaturateOnIntegerOverflow=on  OutDataTypeStr=Inherit: Same as input  ParamDataTypeStr=Inherit: Same as input
  Speed of Sound : Outport  PortDimensions=1
  Air Density : Outport  Port=2  PortDimensions=1
  wires:
  g/(L*R)/1 -> "(T/T0)^(g/LR) "/2
  Height/1 -> Limit altitude  to troposhere/1, Sum/2
  Limit altitude  to troposhere/1 -> Lapse Rate/1
  Product/1 -> rho0/1
  "(T/T0)^(g/LR) "/1 -> Product/1
  1/T0/1 -> "(T/T0)^(g/LR) "/1, Product/2
  gamma*R/1 -> a/1
  a/1 -> Speed of Sound/1
  Sum1/1 -> gamma*R/1, 1/T0/1, Product1/1
  Lapse Rate/1 -> Sum1/2
  Sea Level Temperature/1 -> Sum1/1
  rho0/1 -> Product3/1
  Product3/1 -> Air Density/1
  Stratosphere Model/1 -> Product3/2
  g/R/1 -> Product1/2
  Product1/1 -> Stratosphere Model/1
  Altitude of Troposphere/1 -> Sum/1
  Sum/1 -> Limit altitude  to Stratosphere/1
  Limit altitude  to Stratosphere/1 -> g/R/1

== system AFDNFSmodelSPA/Nonlinear Flight Simulator/Forces and Moments/Aerodynamic Forces and /Aero Attributes/Velocity Magnitude ==
  Velocity : Inport
  Dot Product : DotProduct  InputSameDT=on  OutDataTypeStr=Inherit: Inherit via internal rule
  Sqrt : Sqrt  SaturateOnIntegerOverflow=on
  Velocity Magnitude : Outport
  wires:
  Sqrt/1 -> Velocity Magnitude/1  "abs(V)"
  Velocity/1 -> Dot Product/2, Dot Product/1
  Dot Product/1 -> Sqrt/1

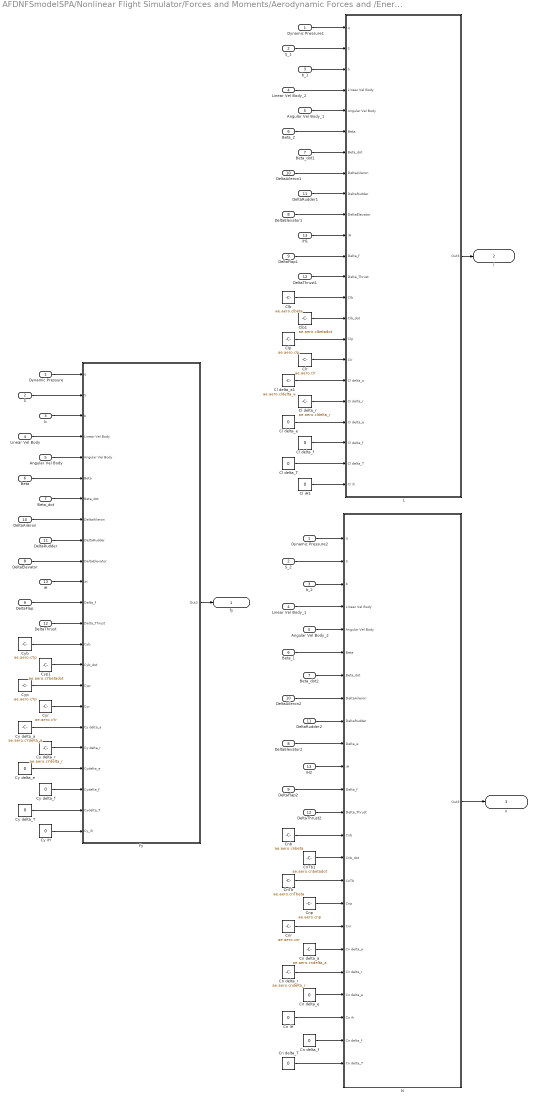
== system AFDNFSmodelSPA/Nonlinear Flight Simulator/Forces and Moments/Aerodynamic Forces and /Energy Analysis1/Lateral-Directional1 ==
  Dynamic Pressure : Inport
  S : Inport  Port=2
  b : Inport  Port=3
  Linear Vel Body : Inport  Port=4
  Angular Vel Body : Inport  Port=5
  Beta : Inport  Port=6
  Beta_dot : Inport  Port=7
  DeltaElevator : Inport  Port=8
  DeltaFlap : Inport  Port=9
  DeltaAileron : Inport  Port=10
  DeltaRudder : Inport  Port=11
  DeltaThrust : Inport  Port=12
  iH : Inport  Port=13
  Angular Vel Body_1 : InportShadow  Port=5
  Angular Vel Body_2 : InportShadow  Port=5
  Beta_1 : InportShadow  Port=6
  Beta_2 : InportShadow  Port=6
  Beta_dot1 : InportShadow  Port=7
  Beta_dot2 : InportShadow  Port=7
  Cl delta_T : Constant  Value=0
  Cl delta_a1 : Constant  Value=ae.aero.cldelta_a
  Cl delta_e : Constant  Value=0
  Cl delta_f : Constant  Value=0
  Cl delta_r : Constant  Value=ae.aero.cldelta_r
  Cl iH1 : Constant  Value=0
  Clb : Constant  Value=ae.aero.clbeta
  Clb1 : Constant  Value=ae.aero.clbetadot
  Clp : Constant  Value=ae.aero.clp
  Clr : Constant  Value=ae.aero.clr
  Cn delta_T : Constant  Value=0
  Cn delta_a : Constant  Value=ae.aero.cndelta_a
  Cn delta_e : Constant  Value=0
  Cn delta_f : Constant  Value=0
  Cn delta_r : Constant  Value=ae.aero.cndelta_r
  Cn iH : Constant  Value=0
  CnTb : Constant  Value=ae.aero.cnTbeta
  CnTb1 : Constant  Value=ae.aero.cnbetadot
  Cnb : Constant  Value=ae.aero.cnbeta
  Cnp : Constant  Value=ae.aero.cnp
  Cnr : Constant  Value=ae.aero.cnr
  Cy delta_T : Constant  Value=0
  Cy delta_a : Constant  Value=ae.aero.cYdelta_a
  Cy delta_e : Constant  Value=0
  Cy delta_f : Constant  Value=0
  Cy delta_r : Constant  Value=ae.aero.cYdelta_r
  Cy iH : Constant  Value=0
  Cyb : Constant  Value=ae.aero.cYp
  Cyp : Constant  Value=ae.aero.cYp
  Cyp1 : Constant  Value=ae.aero.cYbetadot
  Cyr : Constant  Value=ae.aero.cYr
  DeltaAileron1 : InportShadow  Port=10
  DeltaAileron2 : InportShadow  Port=10
  DeltaElevator1 : InportShadow  Port=8
  DeltaElevator2 : InportShadow  Port=8
  DeltaFlap1 : InportShadow  Port=9
  DeltaFlap2 : InportShadow  Port=9
  DeltaRudder1 : InportShadow  Port=11
  DeltaRudder2 : InportShadow  Port=11
  DeltaThrust1 : InportShadow  Port=12
  DeltaThrust2 : InportShadow  Port=12
  Dynamic Pressure1 : InportShadow
  Dynamic Pressure2 : InportShadow
  Fy : Subsystem
  L : Subsystem
  Linear Vel Body_1 : InportShadow  Port=4
  Linear Vel Body_2 : InportShadow  Port=4
  N : Subsystem
  S_1 : InportShadow  Port=2
  S_2 : InportShadow  Port=2
  b_1 : InportShadow  Port=3
  b_2 : InportShadow  Port=3
  iH1 : InportShadow  Port=13
  iH2 : InportShadow  Port=13
  fy : Outport
  l : Outport  Port=2
  n : Outport  Port=3
  wires:
  L/1(Out3) -> l/1
  N/1(Out3) -> n/1
  Fy/1(Out3) -> fy/1
  Dynamic Pressure/1 -> Fy/1(q)
  S/1 -> Fy/2(S)
  b/1 -> Fy/3(b)
  Linear Vel Body/1 -> Fy/4(Linear Vel Body)
  Angular Vel Body/1 -> Fy/5(Angular Vel Body)
  Beta/1 -> Fy/6(Beta)
  Beta_dot/1 -> Fy/7(Beta_dot)
  DeltaAileron/1 -> Fy/8(DeltaAileron)
  DeltaRudder/1 -> Fy/9(DeltaRudder)
  iH/1 -> Fy/11(iH)
  DeltaElevator/1 -> Fy/10(DeltaElevator)
  DeltaFlap/1 -> Fy/12(Delta_f)
  DeltaThrust/1 -> Fy/13(Delta_Thrust)
  DeltaRudder2/1 -> N/9(DeltaRudder)
  DeltaAileron2/1 -> N/8(DeltaAileron)
  Dynamic Pressure2/1 -> N/1(q)
  DeltaThrust2/1 -> N/13(Delta_Thrust)
  b_2/1 -> N/3(b)
  Angular Vel Body_2/1 -> N/5(Angular Vel Body)
  Linear Vel Body_1/1 -> N/4(Linear Vel Body)
  iH2/1 -> N/11(iH)
  Beta_dot2/1 -> N/7(Beta_dot)
  S_2/1 -> N/2(S)
  DeltaElevator2/1 -> N/10(Delta_e)
  DeltaFlap2/1 -> N/12(Delta_f)
  Beta_1/1 -> N/6(Beta)
  Cyb/1 -> Fy/14(Cyb)
  Cyp/1 -> Fy/16(Cyp)
  Cyr/1 -> Fy/17(Cyr)
  Cy delta_a/1 -> Fy/18(Cy delta_a)
  Cy delta_r/1 -> Fy/19(Cy delta_r)
  Cy delta_e/1 -> Fy/20(Cydelta_e)
  Cy delta_f/1 -> Fy/21(Cydelta_f)
  Cy delta_T/1 -> Fy/22(Cydelta_T)
  Cy iH/1 -> Fy/23(Cy_ih)
  Cnb/1 -> N/14(Cnb)
  Cnp/1 -> N/17(Cnp)
  Cn delta_T/1 -> N/24(Cn delta_T)
  CnTb/1 -> N/16(CnTb)
  Cn delta_a/1 -> N/19(Cn delta_a)
  Cn delta_e/1 -> N/21(Cn delta_e)
  Cn delta_r/1 -> N/20(Cn delta_r)
  Cn iH/1 -> N/22(Cn ih)
  Cn delta_f/1 -> N/23(Cn delta_f)
  Cnr/1 -> N/18(Cnr)
  Clb/1 -> L/14(Clb)
  Clp/1 -> L/16(Clp)
  Cl delta_a1/1 -> L/18(Cl delta_a)
  b_1/1 -> L/3(b)
  Dynamic Pressure1/1 -> L/1(q)
  Angular Vel Body_1/1 -> L/5(Angular Vel Body)
  iH1/1 -> L/11(iH)
  DeltaRudder1/1 -> L/9(DeltaRudder)
  DeltaThrust1/1 -> L/13(Delta_Thrust)
  Beta_dot1/1 -> L/7(Beta_dot)
  Beta_2/1 -> L/6(Beta)
  DeltaAileron1/1 -> L/8(DeltaAileron)
  DeltaFlap1/1 -> L/12(Delta_f)
  DeltaElevator1/1 -> L/10(DeltaElevator)
  Linear Vel Body_2/1 -> L/4(Linear Vel Body)
  S_1/1 -> L/2(S)
  Clr/1 -> L/17(Clr)
  Cl delta_e/1 -> L/20(Cl delta_e)
  Cl delta_T/1 -> L/22(Cl delta_T)
  Cl delta_f/1 -> L/21(Cl delta_f)
  Cl delta_r/1 -> L/19(Cl delta_r)
  Cl iH1/1 -> L/23(Cl ih)
  Clb1/1 -> L/15(Clb_dot)
  CnTb1/1 -> N/15(Cnb_dot)
  Cyp1/1 -> Fy/15(Cyb_dot)
